simulink model "example_daqp"  (Simulink 10.2)
settings: Solver=VariableStepAuto  StartTime=0.0  StopTime=10.0  RelTol=1e-3
undefined symbols (not defined in the file or in its folder): dim_daqp
settings Model: Creator=Chr_S  LastModifiedBy=Sc
settings DataIOCC: SaveFormat=Dataset  SignalLoggingSaveFormat=Dataset  ReturnWorkspaceOutputs=on
settings OptimizationCC: LifeSpan=auto
settings DebuggingCC: UnderspecifiedInitializationDetection=Simplified  MergeDetectMultiDrivingBlocksExec=error  FcnCallInpInsideContextMsg=error  SFUnexpectedBacktrackingDiag=error  SFNoUnconditionalDefaultTransitionDiag=error  SFExecutionAtInitializationDiag=warning
settings HardwareCC: ProdBitPerPointer=64  ProdBitPerSizeT=64  ProdBitPerPtrDiffT=64  ProdLargestAtomicFloat=Float  ProdIntDivRoundTo=Zero  ProdEndianess=LittleEndian  ProdWordSize=64  ProdHWDeviceType=Intel->x86-64 (Windows64)
settings ModelReferenceCC: PropagateSignalLabelsOutOfModel=on
settings SFSimCC: SimUseLocalCustomCode=on
settings RTWCC: RTWUseLocalCustomCode=on
settings GRTTargetCC: TargetLangStandard=C99 (ISO)  CombineOutputUpdateFcns=on  GRTInterface=off
settings ConfigComp: CovMetricSettings=dwe  CovSaveCumulativeToWorkspaceVar=off  CovSaveSingleToWorkspaceVar=off  CovExternalEMLEnable=on

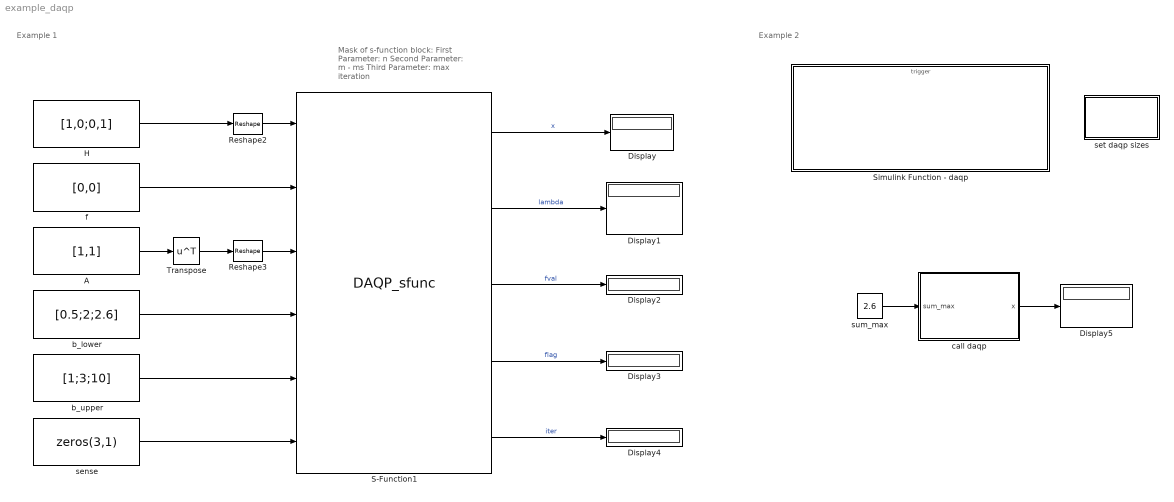
== system example_daqp ==
  note: Example 2
  note: Example 1
  note: Mask of s-function block:
      | First Parameter: n
      | Second Parameter: m - ms
      | Third Parameter: max iteration
  A : Constant  Value=[1,1]
  Display{,1..5} (6 alike) : Display
  H : Constant  Value=[1,0;0,1]
  Reshape2 : Reshape
  Reshape3 : Reshape
  S-Function1 : S-Function  FunctionName=DAQP_sfunc  Parameters=2,1,100  SFunctionDeploymentMode=off  EnableBusSupport=off
  Simulink Function - daqp : Subsystem  TreatAsAtomicUnit=on
  Transpose : Math  Operator=transpose  SaturateOnIntegerOverflow=on
  b_lower : Constant  Value=[0.5;2;2.6]
  b_upper : Constant  Value=[1;3;10]
  call daqp : MATLAB Function  TreatAsAtomicUnit=on
  f : Constant  Value=[0,0]
  sense : Constant  Value=zeros(3,1)
  set daqp sizes : Subsystem  mask(Create a struct "dim_daqp" in workspace){n=2, m=3, ms=2}
      mask prompts: n "Number of decision variables"; m "Number of constraints (general + simple)"; ms "Number of simple bounds"
      mask init:
      | assignin('base','dim_daqp',struct('n',n,'m',m,'ms',ms));
      mask Display: fprintf('n = %d\nm = %d\nms = %d',n,m,ms);
  sum_max : Constant  Value=2.6
  wires:
  S-Function1/1 -> Display/1  "x"
  S-Function1/2 -> Display1/1  "lambda"
  Reshape3/1 -> S-Function1/3
  sense/1 -> S-Function1/6
  b_lower/1 -> S-Function1/4
  b_upper/1 -> S-Function1/5
  H/1 -> Reshape2/1
  A/1 -> Transpose/1
  Reshape2/1 -> S-Function1/1
  f/1 -> S-Function1/2
  Transpose/1 -> Reshape3/1
  S-Function1/3 -> Display2/1  "fval"
  S-Function1/4 -> Display3/1  "flag"
  S-Function1/5 -> Display4/1  "iter"
  call daqp/1(x) -> Display5/1
  sum_max/1 -> call daqp/1(sum_max)

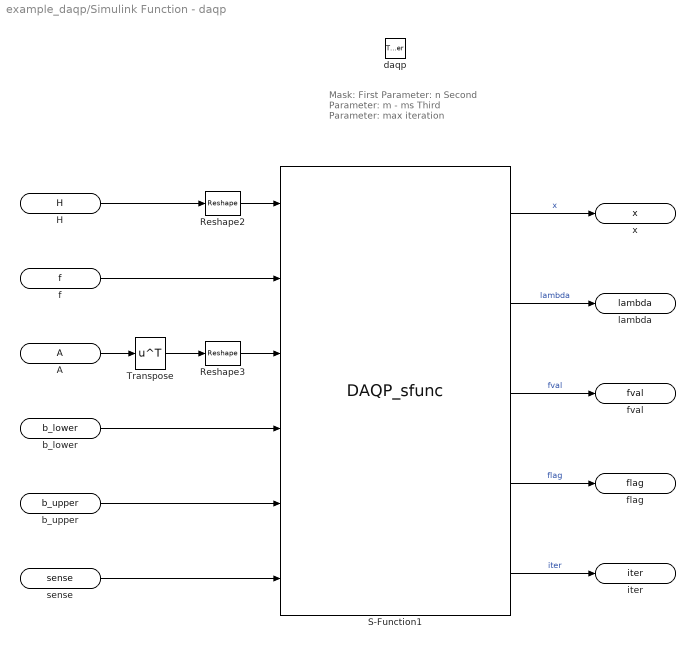
== system example_daqp/Simulink Function - daqp ==
  note: Mask:
      | First Parameter: n
      | Second Parameter: m - ms
      | Third Parameter: max iteration
  daqp : TriggerPort  TriggerType=function-call  IsSimulinkFunction=on  FunctionName=daqp  FunctionVisibility=scoped  VariantControl=(inherit)
  Reshape2 : Reshape
  Reshape3 : Reshape
  S-Function1 : S-Function  FunctionName=DAQP_sfunc  Parameters=dim_daqp.n,dim_daqp.m-dim_daqp.ms,100  SFunctionDeploymentMode=off  EnableBusSupport=off
  Transpose : Math  Operator=transpose  SaturateOnIntegerOverflow=on
  H : ArgIn  DisableCoverage=on  PortDimensions=[dim_daqp.n,dim_daqp.n]  ArgumentName=H
  f : ArgIn  DisableCoverage=on  Port=2  PortDimensions=[dim_daqp.n]  ArgumentName=f
  A : ArgIn  DisableCoverage=on  Port=3  PortDimensions=[dim_daqp.m-dim_daqp.ms,dim_daqp.n]  ArgumentName=A
  b_lower : ArgIn  DisableCoverage=on  Port=4  PortDimensions=[dim_daqp.m]  ArgumentName=b_lower
  b_upper : ArgIn  DisableCoverage=on  Port=5  PortDimensions=[dim_daqp.m]  ArgumentName=b_upper
  sense : ArgIn  DisableCoverage=on  Port=6  PortDimensions=[dim_daqp.m]  ArgumentName=sense
  x : ArgOut  DisableCoverage=on  PortDimensions=[dim_daqp.n]  ArgumentName=x
  lambda : ArgOut  DisableCoverage=on  Port=2  PortDimensions=[dim_daqp.m-dim_daqp.ms]  ArgumentName=lambda
  fval : ArgOut  DisableCoverage=on  Port=3  ArgumentName=fval
  flag : ArgOut  DisableCoverage=on  Port=4  ArgumentName=flag
  iter : ArgOut  DisableCoverage=on  Port=5  ArgumentName=iter
  wires:
  Transpose/1 -> Reshape3/1
  H/1 -> Reshape2/1
  f/1 -> S-Function1/2
  Reshape3/1 -> S-Function1/3
  Reshape2/1 -> S-Function1/1
  S-Function1/1 -> x/1  "x"
  A/1 -> Transpose/1
  S-Function1/2 -> lambda/1  "lambda"
  S-Function1/3 -> fval/1  "fval"
  S-Function1/4 -> flag/1  "flag"
  S-Function1/5 -> iter/1  "iter"
  b_lower/1 -> S-Function1/4
  b_upper/1 -> S-Function1/5
  sense/1 -> S-Function1/6

== system example_daqp/set daqp sizes ==

== matlab function call daqp ==
  data: sum_max input double; x output double
function x = fcn(sum_max)

% Simple qp:
% cost = 0.5* x1^2 + x2^2 
% s.t. 0.5 < x1    < inf
%      2   < x2    < inf
%  sum_max < x1+x2 < inf

H = [1,0;0,1];
f = [0;0];
A = [1,1];
b_lower = [0.5;2;sum_max];
b_upper = [inf;inf;inf];
sense = [0;0;0];


[x,lambda,fval,flag,iter] = daqp(H,f,A,b_lower,b_upper,sense);
